simulink model "QuadcopterControl"  (R2026a)
settings: Solver=VariableStepAuto  StopTime=20
libraries: slpidlib x6, matrix_library x4
settings Model: SimulationMode=accelerator  Creator=nfrey  LastModifiedBy=nfrey
settings DataIOCC: InspectSignalLogs=on

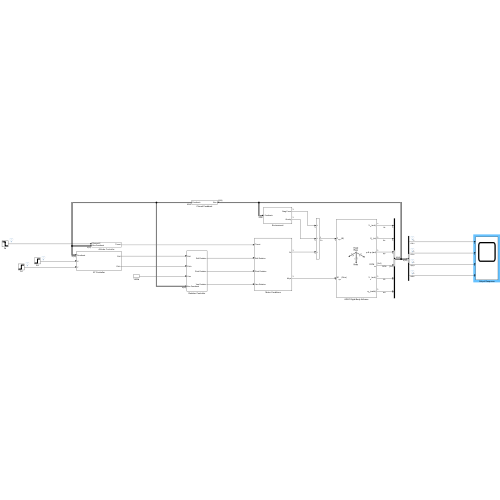
[thumbnail: Simulink's stored preview of the top-level diagram]
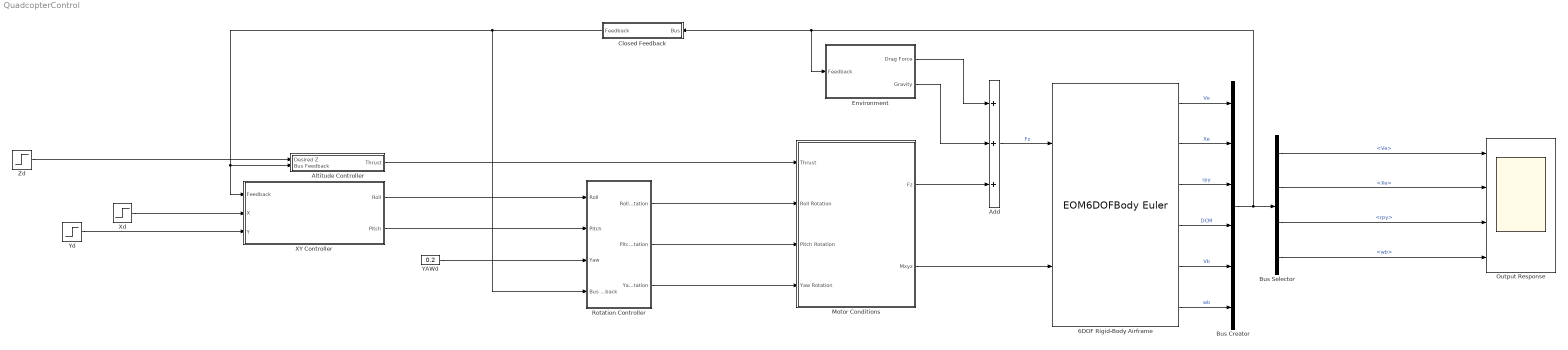
== system QuadcopterControl ==
  6DOF Rigid-Body Airframe : EOM6DOFBodyEuler
  Add : Sum  Inputs=+++
  Altitude Controller : Subsystem
  Bus Creator : BusCreator  Inputs=6
  Bus Selector : BusSelector  OutputSignals=Ve,Xe,rpy,wb
  Closed Feedback : Subsystem
  Environment : Subsystem
  Motor Conditions : Subsystem
  Output Response : Scope  NumInputPorts=4
      settings: ActiveDisplayYMinimum=-17.054653965110973  ActiveDisplayYMaximum=83.725752230949269
  Rotation Controller : Subsystem
  XY Controller : Subsystem
  Xd : Step  FinalValue=10  SampleTime=0
  YAWd : Constant  Value=0.2
  Yd : Step  FinalValue=5  SampleTime=0
  Zd : Step  FinalValue=-10  SampleTime=0
  wires:
  XY Controller/2(Pitch) -> Rotation Controller/2(Pitch)
  XY Controller/1(Roll) -> Rotation Controller/1(Roll)
  YAWd/1 -> Rotation Controller/3(Yaw)
  Bus Selector/3 -> Output Response/3  "<rpy>"
  Motor Conditions/1(Fz) -> Add/3
  Bus Selector/4 -> Output Response/4  "<wb>"
  Rotation Controller/2(Pitch Rotation) -> Motor Conditions/3(Pitch Rotation)
  Rotation Controller/3(Yaw Rotation) -> Motor Conditions/4(Yaw Rotation)
  Altitude Controller/1(Thrust) -> Motor Conditions/1(Thrust)
  Environment/1(Drag Force) -> Add/1
  Rotation Controller/1(Roll Rotation) -> Motor Conditions/2(Roll Rotation)
  Bus Selector/2 -> Output Response/2  "<Xe>"
  Bus Selector/1 -> Output Response/1  "<Ve>"
  6DOF Rigid-Body Airframe/2 -> Bus Creator/2  "Xe"
  6DOF Rigid-Body Airframe/4 -> Bus Creator/4  "DCM"
  6DOF Rigid-Body Airframe/1 -> Bus Creator/1  "Ve"
  6DOF Rigid-Body Airframe/3 -> Bus Creator/3  "rpy"
  6DOF Rigid-Body Airframe/6 -> Bus Creator/6  "wb"
  6DOF Rigid-Body Airframe/5 -> Bus Creator/5  "Vb"
  Bus Creator/1 -> Environment/1(" Feedback"), Closed Feedback/1(" Bus"), Bus Selector/1
  Environment/2(Gravity) -> Add/2
  Motor Conditions/2(Mxyz) -> 6DOF Rigid-Body Airframe/2
  Add/1 -> 6DOF Rigid-Body Airframe/1  "Fz"
  Closed Feedback/1(Feedback) -> Rotation Controller/4(Bus Feedback), XY Controller/1(Feedback), Altitude Controller/2(Bus Feedback)
  Xd/1 -> XY Controller/2(X)
  Yd/1 -> XY Controller/3(Y)
  Zd/1 -> Altitude Controller/1(Desired Z)

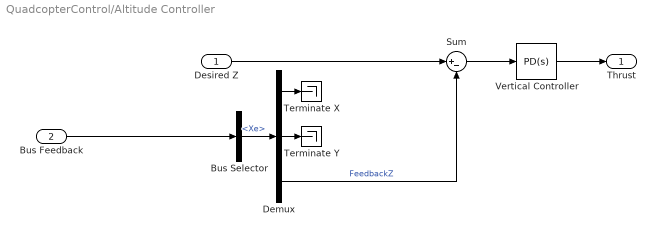
== system QuadcopterControl/Altitude Controller ==
  Desired Z : Inport
  Bus Feedback : Inport  Port=2
  Bus Selector : BusSelector  OutputSignals=Xe
  Demux : Demux  Outputs=3
  Sum : Sum  Inputs=|+-
  Terminate X : Terminator
  Terminate Y : Terminator
  Vertical Controller : slpidlib/PID Controller  Controller=PD  Form=Parallel  TimeDomain=Continuous-time  UseExternalTs=off  SampleTime=-1  IntegratorMethod=Forward Euler  FilterMethod=Forward Euler  ControllerParametersSource=internal  P=1.68756862780495  I=1  UseKiTs=off  D=2.04119632180359  UseExternalDerivativeSource=off  N=476.409993785113  UseFilter=on  TunerSelectOption=Transfer Function Based (PID Tuner App)  InitialConditionSource=internal  InitialConditionForIntegrator=0  InitialConditionForFilter=0  DifferentiatorICPrevScaledInput=0  ExternalReset=none  TrackingMode=off  Kt=1  LimitOutput=off  SatLimitsSource=internal  UpperSaturationLimit=inf  LowerSaturationLimit=-inf  LinearizeAsGain=on  AntiWindupMode=none  Kb=1  LimitIntegrator=off  UpperIntegratorSaturationLimit=inf  LowerIntegratorSaturationLimit=-inf  POutMin=[]  POutMax=[]  IOutMin=[]  IOutMax=[]  DOutMin=[]  DOutMax=[]  NOutMin=[]  NOutMax=[]  SumOutMin=[]  SumOutMax=[]  SaturationOutMin=[]  SaturationOutMax=[]  PParamMin=[]  PParamMax=[]  IParamMin=[]  IParamMax=[]  DParamMin=[]  DParamMax=[]  NParamMin=[]  NParamMax=[]  KbParamMin=[]  KbParamMax=[]  KtParamMin=[]  KtParamMax=[]  KbOutMin=[]  KbOutMax=[]  KtOutMin=[]  KtOutMax=[]  IntegratorOutMin=[]  IntegratorOutMax=[]  FilterOutMin=[]  FilterOutMax=[]  SumI1OutMin=[]  SumI1OutMax=[]  SumI2OutMin=[]  SumI2OutMax=[]  SumI3OutMin=[]  SumI3OutMax=[]  SumI4OutMin=[]  SumI4OutMax=[]  SumDOutMin=[]  SumDOutMax=[]  DifferentiatorOutMin=[]  DifferentiatorOutMax=[]  FilterDiffOutCoefMin=[]  FilterDiffOutCoefMax=[]  ReciprocalOutMin=[]  ReciprocalOutMax=[]  SumDenOutMin=[]  SumDenOutMax=[]  SumNumOutMin=[]  SumNumOutMax=[]  DivideOutMin=[]  DivideOutMax=[]  UdiffTsProdOutMin=[]  UdiffTsProdOutMax=[]  NTsProdOutMin=[]  NTsProdOutMax=[]  UintegralTsProdOutMin=[]  UintegralTsProdOutMax=[]  UngainTsProdOutMin=[]  UngainTsProdOutMax=[]  ClampingZeroOutDataTypeStr=Inherit: Inherit via back propagation  ClampingZeroOutMin=[]  ClampingZeroOutMax=[]  FilterDenConstantOutDataTypeStr=Inherit: Inherit via back propagation  FilterDenConstantOutMin=[]  FilterDenConstantOutMax=[]  PCopyOutDataTypeStr=Inherit: Inherit via back propagation  PCopyOutMin=[]  PCopyOutMax=[]  NCopyOutDataTypeStr=Inherit: Inherit via back propagation  NCopyOutMin=[]  NCopyOutMax=[]  IntegratorContinuousStateAttributes=''  IntegratorStateMustResolveToSignalObject=off  IntegratorRTWStateStorageClass=Auto  FilterContinuousStateAttributes=''  FilterStateMustResolveToSignalObject=off  FilterRTWStateStorageClass=Auto  ParallelPVariant=InternalParameters  IdealPVariant=Disabled  IVariant=Disabled  DVariant=InternalParameters  IntegratorVariant=Disabled  SatVariant=Disabled  AWVariant=Disabled  PCopyVariant=Disabled  TRVariant=Disabled  FdbkBlocksVariant=Forward  IdealPFdbkVariant=Disabled  SatFdbkVariant=Disabled  DerivativeFilterVariant=ContFilter  NVariant=InternalParameters  NCopyVariant=Disabled  FilterICVariant=InternalICsFilter  IntegratorICVariant=Disabled  ExternalResetVariant=Disabled  TRSumVariant=Passthrough  SumFdbkVariant=Disabled  SumVariant=Sum_PD  TsampFilterVariant=InternalTs  TsampNgainVariant=Passthrough  TsampIntegralVariant=Disabled_SignalSpec  ExternalSaturationOutDataTypeStr=Inherit: Same as second input  DerivativeSourceVariant=ErrorSignal  PreIntVariant=InternalPreInt
  Thrust : Outport
  wires:
  Bus Feedback/1 -> Bus Selector/1
  Bus Selector/1 -> Demux/1  "<Xe>"
  Demux/1 -> Terminate X/1
  Demux/2 -> Terminate Y/1
  Desired Z/1 -> Sum/1
  Demux/3 -> Sum/2  "FeedbackZ"
  Sum/1 -> Vertical Controller/1
  Vertical Controller/1 -> Thrust/1

== system QuadcopterControl/Closed Feedback ==
  " Bus" : Inport
  Feedback : Outport
  wires:
  " Bus"/1 -> Feedback/1

== system QuadcopterControl/Environment ==
  " Feedback" : Inport
  Drag : Subsystem
  Gravity Variable : Subsystem
  Drag Force : Outport
  Gravity : Outport  Port=2
  wires:
  " Feedback"/1 -> Gravity Variable/1(In1), Drag/1(In1)
  Drag/1(Drag Force) -> Drag Force/1
  Gravity Variable/1(Gravity) -> Gravity/1

== system QuadcopterControl/Motor Conditions ==
  Thrust : Inport
  Roll Rotation : Inport  Port=2
  Pitch Rotation : Inport  Port=3
  Yaw Rotation : Inport  Port=4
  Moment & Net Force : Subsystem
  Rotor Correction : Subsystem
  Fz : Outport
  Mxyz : Outport  Port=2
  wires:
  Roll Rotation/1 -> Rotor Correction/2(Roll)
  Rotor Correction/1(Propeller Velocity) -> Moment & Net Force/1(Propeller Velocity)
  Moment & Net Force/1(OutputFz) -> Fz/1
  Pitch Rotation/1 -> Rotor Correction/3(Pitch)
  Thrust/1 -> Rotor Correction/1(Thrust)
  Moment & Net Force/2(Moment) -> Mxyz/1
  Yaw Rotation/1 -> Rotor Correction/4(Yaw)

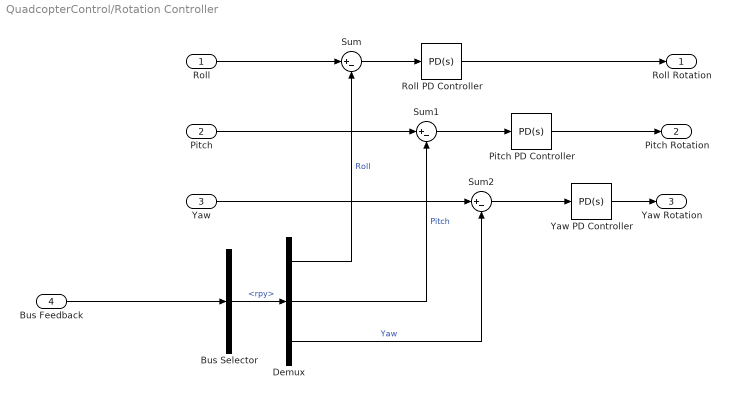
== system QuadcopterControl/Rotation Controller ==
  Roll : Inport
  Pitch : Inport  Port=2
  Yaw : Inport  Port=3
  Bus Feedback : Inport  Port=4
  Bus Selector : BusSelector  OutputSignals=rpy
  Demux : Demux  Outputs=3
  Pitch PD Controller : slpidlib/PID Controller  Controller=PD  Form=Parallel  TimeDomain=Continuous-time  UseExternalTs=off  SampleTime=-1  IntegratorMethod=Forward Euler  FilterMethod=Forward Euler  ControllerParametersSource=internal  P=.684  I=1  UseKiTs=off  D=1.41  UseExternalDerivativeSource=off  N=100  UseFilter=on  TunerSelectOption=Transfer Function Based (PID Tuner App)  InitialConditionSource=internal  InitialConditionForIntegrator=0  InitialConditionForFilter=0  DifferentiatorICPrevScaledInput=0  ExternalReset=none  TrackingMode=off  Kt=1  LimitOutput=off  SatLimitsSource=internal  UpperSaturationLimit=inf  LowerSaturationLimit=-inf  LinearizeAsGain=on  AntiWindupMode=none  Kb=1  LimitIntegrator=off  UpperIntegratorSaturationLimit=inf  LowerIntegratorSaturationLimit=-inf  POutMin=[]  POutMax=[]  IOutMin=[]  IOutMax=[]  DOutMin=[]  DOutMax=[]  NOutMin=[]  NOutMax=[]  SumOutMin=[]  SumOutMax=[]  SaturationOutMin=[]  SaturationOutMax=[]  PParamMin=[]  PParamMax=[]  IParamMin=[]  IParamMax=[]  DParamMin=[]  DParamMax=[]  NParamMin=[]  NParamMax=[]  KbParamMin=[]  KbParamMax=[]  KtParamMin=[]  KtParamMax=[]  KbOutMin=[]  KbOutMax=[]  KtOutMin=[]  KtOutMax=[]  IntegratorOutMin=[]  IntegratorOutMax=[]  FilterOutMin=[]  FilterOutMax=[]  SumI1OutMin=[]  SumI1OutMax=[]  SumI2OutMin=[]  SumI2OutMax=[]  SumI3OutMin=[]  SumI3OutMax=[]  SumI4OutMin=[]  SumI4OutMax=[]  SumDOutMin=[]  SumDOutMax=[]  DifferentiatorOutMin=[]  DifferentiatorOutMax=[]  FilterDiffOutCoefMin=[]  FilterDiffOutCoefMax=[]  ReciprocalOutMin=[]  ReciprocalOutMax=[]  SumDenOutMin=[]  SumDenOutMax=[]  SumNumOutMin=[]  SumNumOutMax=[]  DivideOutMin=[]  DivideOutMax=[]  UdiffTsProdOutMin=[]  UdiffTsProdOutMax=[]  NTsProdOutMin=[]  NTsProdOutMax=[]  UintegralTsProdOutMin=[]  UintegralTsProdOutMax=[]  UngainTsProdOutMin=[]  UngainTsProdOutMax=[]  ClampingZeroOutDataTypeStr=Inherit: Inherit via back propagation  ClampingZeroOutMin=[]  ClampingZeroOutMax=[]  FilterDenConstantOutDataTypeStr=Inherit: Inherit via back propagation  FilterDenConstantOutMin=[]  FilterDenConstantOutMax=[]  PCopyOutDataTypeStr=Inherit: Inherit via back propagation  PCopyOutMin=[]  PCopyOutMax=[]  NCopyOutDataTypeStr=Inherit: Inherit via back propagation  NCopyOutMin=[]  NCopyOutMax=[]  IntegratorContinuousStateAttributes=''  IntegratorStateMustResolveToSignalObject=off  IntegratorRTWStateStorageClass=Auto  FilterContinuousStateAttributes=''  FilterStateMustResolveToSignalObject=off  FilterRTWStateStorageClass=Auto  ParallelPVariant=InternalParameters  IdealPVariant=Disabled  IVariant=Disabled  DVariant=InternalParameters  IntegratorVariant=Disabled  SatVariant=Disabled  AWVariant=Disabled  PCopyVariant=Disabled  TRVariant=Disabled  FdbkBlocksVariant=Forward  IdealPFdbkVariant=Disabled  SatFdbkVariant=Disabled  DerivativeFilterVariant=ContFilter  NVariant=InternalParameters  NCopyVariant=Disabled  FilterICVariant=InternalICsFilter  IntegratorICVariant=Disabled  ExternalResetVariant=Disabled  TRSumVariant=Passthrough  SumFdbkVariant=Disabled  SumVariant=Sum_PD  TsampFilterVariant=InternalTs  TsampNgainVariant=Passthrough  TsampIntegralVariant=Disabled_SignalSpec  ExternalSaturationOutDataTypeStr=Inherit: Same as second input  DerivativeSourceVariant=ErrorSignal  PreIntVariant=InternalPreInt
  Roll PD Controller : slpidlib/PID Controller  Controller=PD  Form=Parallel  TimeDomain=Continuous-time  UseExternalTs=off  SampleTime=-1  IntegratorMethod=Forward Euler  FilterMethod=Forward Euler  ControllerParametersSource=internal  P=.684  I=1  UseKiTs=off  D=1.41  UseExternalDerivativeSource=off  N=100  UseFilter=on  TunerSelectOption=Transfer Function Based (PID Tuner App)  InitialConditionSource=internal  InitialConditionForIntegrator=0  InitialConditionForFilter=0  DifferentiatorICPrevScaledInput=0  ExternalReset=none  TrackingMode=off  Kt=1  LimitOutput=off  SatLimitsSource=internal  UpperSaturationLimit=inf  LowerSaturationLimit=-inf  LinearizeAsGain=on  AntiWindupMode=none  Kb=1  LimitIntegrator=off  UpperIntegratorSaturationLimit=inf  LowerIntegratorSaturationLimit=-inf  POutMin=[]  POutMax=[]  IOutMin=[]  IOutMax=[]  DOutMin=[]  DOutMax=[]  NOutMin=[]  NOutMax=[]  SumOutMin=[]  SumOutMax=[]  SaturationOutMin=[]  SaturationOutMax=[]  PParamMin=[]  PParamMax=[]  IParamMin=[]  IParamMax=[]  DParamMin=[]  DParamMax=[]  NParamMin=[]  NParamMax=[]  KbParamMin=[]  KbParamMax=[]  KtParamMin=[]  KtParamMax=[]  KbOutMin=[]  KbOutMax=[]  KtOutMin=[]  KtOutMax=[]  IntegratorOutMin=[]  IntegratorOutMax=[]  FilterOutMin=[]  FilterOutMax=[]  SumI1OutMin=[]  SumI1OutMax=[]  SumI2OutMin=[]  SumI2OutMax=[]  SumI3OutMin=[]  SumI3OutMax=[]  SumI4OutMin=[]  SumI4OutMax=[]  SumDOutMin=[]  SumDOutMax=[]  DifferentiatorOutMin=[]  DifferentiatorOutMax=[]  FilterDiffOutCoefMin=[]  FilterDiffOutCoefMax=[]  ReciprocalOutMin=[]  ReciprocalOutMax=[]  SumDenOutMin=[]  SumDenOutMax=[]  SumNumOutMin=[]  SumNumOutMax=[]  DivideOutMin=[]  DivideOutMax=[]  UdiffTsProdOutMin=[]  UdiffTsProdOutMax=[]  NTsProdOutMin=[]  NTsProdOutMax=[]  UintegralTsProdOutMin=[]  UintegralTsProdOutMax=[]  UngainTsProdOutMin=[]  UngainTsProdOutMax=[]  ClampingZeroOutDataTypeStr=Inherit: Inherit via back propagation  ClampingZeroOutMin=[]  ClampingZeroOutMax=[]  FilterDenConstantOutDataTypeStr=Inherit: Inherit via back propagation  FilterDenConstantOutMin=[]  FilterDenConstantOutMax=[]  PCopyOutDataTypeStr=Inherit: Inherit via back propagation  PCopyOutMin=[]  PCopyOutMax=[]  NCopyOutDataTypeStr=Inherit: Inherit via back propagation  NCopyOutMin=[]  NCopyOutMax=[]  IntegratorContinuousStateAttributes=''  IntegratorStateMustResolveToSignalObject=off  IntegratorRTWStateStorageClass=Auto  FilterContinuousStateAttributes=''  FilterStateMustResolveToSignalObject=off  FilterRTWStateStorageClass=Auto  ParallelPVariant=InternalParameters  IdealPVariant=Disabled  IVariant=Disabled  DVariant=InternalParameters  IntegratorVariant=Disabled  SatVariant=Disabled  AWVariant=Disabled  PCopyVariant=Disabled  TRVariant=Disabled  FdbkBlocksVariant=Forward  IdealPFdbkVariant=Disabled  SatFdbkVariant=Disabled  DerivativeFilterVariant=ContFilter  NVariant=InternalParameters  NCopyVariant=Disabled  FilterICVariant=InternalICsFilter  IntegratorICVariant=Disabled  ExternalResetVariant=Disabled  TRSumVariant=Passthrough  SumFdbkVariant=Disabled  SumVariant=Sum_PD  TsampFilterVariant=InternalTs  TsampNgainVariant=Passthrough  TsampIntegralVariant=Disabled_SignalSpec  ExternalSaturationOutDataTypeStr=Inherit: Same as second input  DerivativeSourceVariant=ErrorSignal  PreIntVariant=InternalPreInt
  Sum : Sum  Inputs=|+-
  Sum1 : Sum  Inputs=|+-
  Sum2 : Sum  Inputs=|+-
  Yaw PD Controller : slpidlib/PID Controller  Controller=PD  Form=Parallel  TimeDomain=Continuous-time  UseExternalTs=off  SampleTime=-1  IntegratorMethod=Forward Euler  FilterMethod=Forward Euler  ControllerParametersSource=internal  P=0.684167402629352  I=1  UseKiTs=off  D=1.4072621028923  UseExternalDerivativeSource=off  N=100  UseFilter=on  TunerSelectOption=Transfer Function Based (PID Tuner App)  InitialConditionSource=internal  InitialConditionForIntegrator=0  InitialConditionForFilter=0  DifferentiatorICPrevScaledInput=0  ExternalReset=none  TrackingMode=off  Kt=1  LimitOutput=off  SatLimitsSource=internal  UpperSaturationLimit=inf  LowerSaturationLimit=-inf  LinearizeAsGain=on  AntiWindupMode=none  Kb=1  LimitIntegrator=off  UpperIntegratorSaturationLimit=inf  LowerIntegratorSaturationLimit=-inf  POutMin=[]  POutMax=[]  IOutMin=[]  IOutMax=[]  DOutMin=[]  DOutMax=[]  NOutMin=[]  NOutMax=[]  SumOutMin=[]  SumOutMax=[]  SaturationOutMin=[]  SaturationOutMax=[]  PParamMin=[]  PParamMax=[]  IParamMin=[]  IParamMax=[]  DParamMin=[]  DParamMax=[]  NParamMin=[]  NParamMax=[]  KbParamMin=[]  KbParamMax=[]  KtParamMin=[]  KtParamMax=[]  KbOutMin=[]  KbOutMax=[]  KtOutMin=[]  KtOutMax=[]  IntegratorOutMin=[]  IntegratorOutMax=[]  FilterOutMin=[]  FilterOutMax=[]  SumI1OutMin=[]  SumI1OutMax=[]  SumI2OutMin=[]  SumI2OutMax=[]  SumI3OutMin=[]  SumI3OutMax=[]  SumI4OutMin=[]  SumI4OutMax=[]  SumDOutMin=[]  SumDOutMax=[]  DifferentiatorOutMin=[]  DifferentiatorOutMax=[]  FilterDiffOutCoefMin=[]  FilterDiffOutCoefMax=[]  ReciprocalOutMin=[]  ReciprocalOutMax=[]  SumDenOutMin=[]  SumDenOutMax=[]  SumNumOutMin=[]  SumNumOutMax=[]  DivideOutMin=[]  DivideOutMax=[]  UdiffTsProdOutMin=[]  UdiffTsProdOutMax=[]  NTsProdOutMin=[]  NTsProdOutMax=[]  UintegralTsProdOutMin=[]  UintegralTsProdOutMax=[]  UngainTsProdOutMin=[]  UngainTsProdOutMax=[]  ClampingZeroOutDataTypeStr=Inherit: Inherit via back propagation  ClampingZeroOutMin=[]  ClampingZeroOutMax=[]  FilterDenConstantOutDataTypeStr=Inherit: Inherit via back propagation  FilterDenConstantOutMin=[]  FilterDenConstantOutMax=[]  PCopyOutDataTypeStr=Inherit: Inherit via back propagation  PCopyOutMin=[]  PCopyOutMax=[]  NCopyOutDataTypeStr=Inherit: Inherit via back propagation  NCopyOutMin=[]  NCopyOutMax=[]  IntegratorContinuousStateAttributes=''  IntegratorStateMustResolveToSignalObject=off  IntegratorRTWStateStorageClass=Auto  FilterContinuousStateAttributes=''  FilterStateMustResolveToSignalObject=off  FilterRTWStateStorageClass=Auto  ParallelPVariant=InternalParameters  IdealPVariant=Disabled  IVariant=Disabled  DVariant=InternalParameters  IntegratorVariant=Disabled  SatVariant=Disabled  AWVariant=Disabled  PCopyVariant=Disabled  TRVariant=Disabled  FdbkBlocksVariant=Forward  IdealPFdbkVariant=Disabled  SatFdbkVariant=Disabled  DerivativeFilterVariant=ContFilter  NVariant=InternalParameters  NCopyVariant=Disabled  FilterICVariant=InternalICsFilter  IntegratorICVariant=Disabled  ExternalResetVariant=Disabled  TRSumVariant=Passthrough  SumFdbkVariant=Disabled  SumVariant=Sum_PD  TsampFilterVariant=InternalTs  TsampNgainVariant=Passthrough  TsampIntegralVariant=Disabled_SignalSpec  ExternalSaturationOutDataTypeStr=Inherit: Same as second input  DerivativeSourceVariant=ErrorSignal  PreIntVariant=InternalPreInt
  Roll Rotation : Outport
  Pitch Rotation : Outport  Port=2
  Yaw Rotation : Outport  Port=3
  wires:
  Bus Feedback/1 -> Bus Selector/1
  Bus Selector/1 -> Demux/1  "<rpy>"
  Roll/1 -> Sum/1
  Sum/1 -> Roll PD Controller/1
  Sum1/1 -> Pitch PD Controller/1
  Pitch/1 -> Sum1/1
  Yaw/1 -> Sum2/1
  Sum2/1 -> Yaw PD Controller/1
  Roll PD Controller/1 -> Roll Rotation/1
  Pitch PD Controller/1 -> Pitch Rotation/1
  Yaw PD Controller/1 -> Yaw Rotation/1
  Demux/1 -> Sum/2  "Roll"
  Demux/2 -> Sum1/2  "Pitch"
  Demux/3 -> Sum2/2  "Yaw"

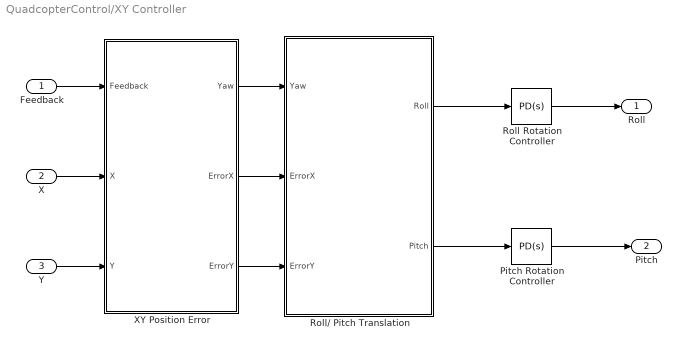
== system QuadcopterControl/XY Controller ==
  Feedback : Inport
  X : Inport  Port=2
  Y : Inport  Port=3
  Pitch Rotation Controller : slpidlib/PID Controller  Controller=PD  Form=Parallel  TimeDomain=Continuous-time  UseExternalTs=off  SampleTime=-1  IntegratorMethod=Forward Euler  FilterMethod=Forward Euler  ControllerParametersSource=internal  P=0.02  I=1  UseKiTs=off  D=0.15  UseExternalDerivativeSource=off  N=170  UseFilter=on  TunerSelectOption=Transfer Function Based (PID Tuner App)  InitialConditionSource=internal  InitialConditionForIntegrator=0  InitialConditionForFilter=0  DifferentiatorICPrevScaledInput=0  ExternalReset=none  TrackingMode=off  Kt=1  LimitOutput=on  SatLimitsSource=internal  UpperSaturationLimit=0.25  LowerSaturationLimit=-0.25  LinearizeAsGain=on  AntiWindupMode=none  Kb=1  LimitIntegrator=off  UpperIntegratorSaturationLimit=inf  LowerIntegratorSaturationLimit=-inf  POutMin=[]  POutMax=[]  IOutMin=[]  IOutMax=[]  DOutMin=[]  DOutMax=[]  NOutMin=[]  NOutMax=[]  SumOutMin=[]  SumOutMax=[]  SaturationOutMin=[]  SaturationOutMax=[]  PParamMin=[]  PParamMax=[]  IParamMin=[]  IParamMax=[]  DParamMin=[]  DParamMax=[]  NParamMin=[]  NParamMax=[]  KbParamMin=[]  KbParamMax=[]  KtParamMin=[]  KtParamMax=[]  KbOutMin=[]  KbOutMax=[]  KtOutMin=[]  KtOutMax=[]  IntegratorOutMin=[]  IntegratorOutMax=[]  FilterOutMin=[]  FilterOutMax=[]  SumI1OutMin=[]  SumI1OutMax=[]  SumI2OutMin=[]  SumI2OutMax=[]  SumI3OutMin=[]  SumI3OutMax=[]  SumI4OutMin=[]  SumI4OutMax=[]  SumDOutMin=[]  SumDOutMax=[]  DifferentiatorOutMin=[]  DifferentiatorOutMax=[]  FilterDiffOutCoefMin=[]  FilterDiffOutCoefMax=[]  ReciprocalOutMin=[]  ReciprocalOutMax=[]  SumDenOutMin=[]  SumDenOutMax=[]  SumNumOutMin=[]  SumNumOutMax=[]  DivideOutMin=[]  DivideOutMax=[]  UdiffTsProdOutMin=[]  UdiffTsProdOutMax=[]  NTsProdOutMin=[]  NTsProdOutMax=[]  UintegralTsProdOutMin=[]  UintegralTsProdOutMax=[]  UngainTsProdOutMin=[]  UngainTsProdOutMax=[]  ClampingZeroOutDataTypeStr=Inherit: Inherit via back propagation  ClampingZeroOutMin=[]  ClampingZeroOutMax=[]  FilterDenConstantOutDataTypeStr=Inherit: Inherit via back propagation  FilterDenConstantOutMin=[]  FilterDenConstantOutMax=[]  PCopyOutDataTypeStr=Inherit: Inherit via back propagation  PCopyOutMin=[]  PCopyOutMax=[]  NCopyOutDataTypeStr=Inherit: Inherit via back propagation  NCopyOutMin=[]  NCopyOutMax=[]  IntegratorContinuousStateAttributes=''  IntegratorStateMustResolveToSignalObject=off  IntegratorRTWStateStorageClass=Auto  FilterContinuousStateAttributes=''  FilterStateMustResolveToSignalObject=off  FilterRTWStateStorageClass=Auto  ParallelPVariant=InternalParameters  IdealPVariant=Disabled  IVariant=Disabled  DVariant=InternalParameters  IntegratorVariant=Disabled  SatVariant=Enabled  AWVariant=Disabled  PCopyVariant=Disabled  TRVariant=Disabled  FdbkBlocksVariant=Forward  IdealPFdbkVariant=Disabled  SatFdbkVariant=Disabled  DerivativeFilterVariant=ContFilter  NVariant=InternalParameters  NCopyVariant=Disabled  FilterICVariant=InternalICsFilter  IntegratorICVariant=Disabled  ExternalResetVariant=Disabled  TRSumVariant=Passthrough  SumFdbkVariant=Disabled  SumVariant=Sum_PD  TsampFilterVariant=InternalTs  TsampNgainVariant=Passthrough  TsampIntegralVariant=Disabled_SignalSpec  ExternalSaturationOutDataTypeStr=Inherit: Same as second input  DerivativeSourceVariant=ErrorSignal  PreIntVariant=InternalPreInt
  Roll Rotation Controller : slpidlib/PID Controller  Controller=PD  Form=Parallel  TimeDomain=Continuous-time  UseExternalTs=off  SampleTime=-1  IntegratorMethod=Forward Euler  FilterMethod=Forward Euler  ControllerParametersSource=internal  P=0.02  I=1  UseKiTs=off  D=0.15  UseExternalDerivativeSource=off  N=170  UseFilter=on  TunerSelectOption=Transfer Function Based (PID Tuner App)  InitialConditionSource=internal  InitialConditionForIntegrator=0  InitialConditionForFilter=0  DifferentiatorICPrevScaledInput=0  ExternalReset=none  TrackingMode=off  Kt=1  LimitOutput=on  SatLimitsSource=internal  UpperSaturationLimit=.25  LowerSaturationLimit=-.25  LinearizeAsGain=on  AntiWindupMode=none  Kb=1  LimitIntegrator=off  UpperIntegratorSaturationLimit=inf  LowerIntegratorSaturationLimit=-inf  POutMin=[]  POutMax=[]  IOutMin=[]  IOutMax=[]  DOutMin=[]  DOutMax=[]  NOutMin=[]  NOutMax=[]  SumOutMin=[]  SumOutMax=[]  SaturationOutMin=[]  SaturationOutMax=[]  PParamMin=[]  PParamMax=[]  IParamMin=[]  IParamMax=[]  DParamMin=[]  DParamMax=[]  NParamMin=[]  NParamMax=[]  KbParamMin=[]  KbParamMax=[]  KtParamMin=[]  KtParamMax=[]  KbOutMin=[]  KbOutMax=[]  KtOutMin=[]  KtOutMax=[]  IntegratorOutMin=[]  IntegratorOutMax=[]  FilterOutMin=[]  FilterOutMax=[]  SumI1OutMin=[]  SumI1OutMax=[]  SumI2OutMin=[]  SumI2OutMax=[]  SumI3OutMin=[]  SumI3OutMax=[]  SumI4OutMin=[]  SumI4OutMax=[]  SumDOutMin=[]  SumDOutMax=[]  DifferentiatorOutMin=[]  DifferentiatorOutMax=[]  FilterDiffOutCoefMin=[]  FilterDiffOutCoefMax=[]  ReciprocalOutMin=[]  ReciprocalOutMax=[]  SumDenOutMin=[]  SumDenOutMax=[]  SumNumOutMin=[]  SumNumOutMax=[]  DivideOutMin=[]  DivideOutMax=[]  UdiffTsProdOutMin=[]  UdiffTsProdOutMax=[]  NTsProdOutMin=[]  NTsProdOutMax=[]  UintegralTsProdOutMin=[]  UintegralTsProdOutMax=[]  UngainTsProdOutMin=[]  UngainTsProdOutMax=[]  ClampingZeroOutDataTypeStr=Inherit: Inherit via back propagation  ClampingZeroOutMin=[]  ClampingZeroOutMax=[]  FilterDenConstantOutDataTypeStr=Inherit: Inherit via back propagation  FilterDenConstantOutMin=[]  FilterDenConstantOutMax=[]  PCopyOutDataTypeStr=Inherit: Inherit via back propagation  PCopyOutMin=[]  PCopyOutMax=[]  NCopyOutDataTypeStr=Inherit: Inherit via back propagation  NCopyOutMin=[]  NCopyOutMax=[]  IntegratorContinuousStateAttributes=''  IntegratorStateMustResolveToSignalObject=off  IntegratorRTWStateStorageClass=Auto  FilterContinuousStateAttributes=''  FilterStateMustResolveToSignalObject=off  FilterRTWStateStorageClass=Auto  ParallelPVariant=InternalParameters  IdealPVariant=Disabled  IVariant=Disabled  DVariant=InternalParameters  IntegratorVariant=Disabled  SatVariant=Enabled  AWVariant=Disabled  PCopyVariant=Disabled  TRVariant=Disabled  FdbkBlocksVariant=Forward  IdealPFdbkVariant=Disabled  SatFdbkVariant=Disabled  DerivativeFilterVariant=ContFilter  NVariant=InternalParameters  NCopyVariant=Disabled  FilterICVariant=InternalICsFilter  IntegratorICVariant=Disabled  ExternalResetVariant=Disabled  TRSumVariant=Passthrough  SumFdbkVariant=Disabled  SumVariant=Sum_PD  TsampFilterVariant=InternalTs  TsampNgainVariant=Passthrough  TsampIntegralVariant=Disabled_SignalSpec  ExternalSaturationOutDataTypeStr=Inherit: Same as second input  DerivativeSourceVariant=ErrorSignal  PreIntVariant=InternalPreInt
  Roll/ Pitch Translation : Subsystem
  XY Position Error : Subsystem
  Roll : Outport
  Pitch : Outport  Port=2
  wires:
  Feedback/1 -> XY Position Error/1(Feedback)
  X/1 -> XY Position Error/2(X)
  Y/1 -> XY Position Error/3(Y)
  XY Position Error/1(Yaw) -> Roll/ Pitch Translation/1(Yaw)
  XY Position Error/2(ErrorX) -> Roll/ Pitch Translation/2(ErrorX)
  XY Position Error/3(ErrorY) -> Roll/ Pitch Translation/3(ErrorY)
  Pitch Rotation Controller/1 -> Pitch/1
  Roll/ Pitch Translation/2(Pitch) -> Pitch Rotation Controller/1
  Roll/ Pitch Translation/1(Roll) -> Roll Rotation Controller/1
  Roll Rotation Controller/1 -> Roll/1

== system QuadcopterControl/Environment/Drag ==
  In1 : Inport
  Bus Selector : BusSelector  OutputSignals=Vb
  Dot Product : DotProduct  OutDataTypeStr=Inherit: Inherit via internal rule
  Drag Gain : Gain  Gain=-0.005
  Product : Product
  Sqrt : Sqrt
  Drag Force : Outport
  wires:
  In1/1 -> Bus Selector/1
  Bus Selector/1 -> Dot Product/1, Product/2, Dot Product/2  "<Vb>"
  Dot Product/1 -> Sqrt/1
  Sqrt/1 -> Product/1
  Product/1 -> Drag Gain/1
  Drag Gain/1 -> Drag Force/1

== system QuadcopterControl/Environment/Gravity Variable ==
  In1 : Inport
  Gravity Acceleration : Subsystem
  Mass : Gain
  Gravity : Outport
  wires:
  Gravity Acceleration/1(Out1) -> Mass/1
  Mass/1 -> Gravity/1
  In1/1 -> Gravity Acceleration/1(In1)

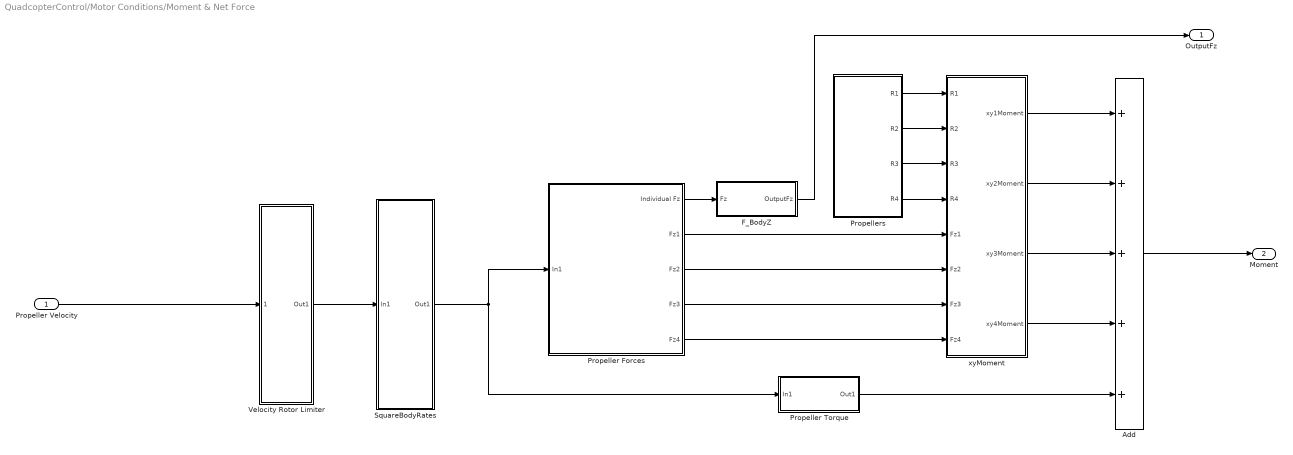
== system QuadcopterControl/Motor Conditions/Moment & Net Force ==
  Propeller Velocity : Inport
  Add : Sum  Inputs=+++++
  F_BodyZ : Subsystem
  Propeller Forces : Subsystem
  "Propeller Torque " : Subsystem
  Propellers : Subsystem
  SquareBodyRates : Subsystem
  Velocity Rotor Limiter : Subsystem
  xyMoment : Subsystem
  OutputFz : Outport
  Moment : Outport  Port=2
  wires:
  Add/1 -> Moment/1
  F_BodyZ/1(OutputFz) -> OutputFz/1
  Propeller Velocity/1 -> Velocity Rotor Limiter/1(Propeller Velocity)
  Propeller Forces/5(Fz4) -> xyMoment/8(Fz4)
  Propeller Forces/4(Fz3) -> xyMoment/7(Fz3)
  Propeller Forces/3(Fz2) -> xyMoment/6(Fz2)
  Propeller Forces/2(Fz1) -> xyMoment/5(Fz1)
  Propellers/4(R4) -> xyMoment/4(R4)
  Propellers/3(R3) -> xyMoment/3(R3)
  Propellers/2(R2) -> xyMoment/2(R2)
  Propellers/1(R1) -> xyMoment/1(R1)
  Propeller Forces/1(Individual Fz) -> F_BodyZ/1(Fz)
  xyMoment/1(xy1Moment) -> Add/1
  xyMoment/2(xy2Moment) -> Add/2
  xyMoment/3(xy3Moment) -> Add/3
  xyMoment/4(xy4Moment) -> Add/4
  "Propeller Torque "/1(Out1) -> Add/5
  SquareBodyRates/1(Out1) -> "Propeller Torque "/1(In1), Propeller Forces/1(In1)
  Velocity Rotor Limiter/1(Out1) -> SquareBodyRates/1(In1)

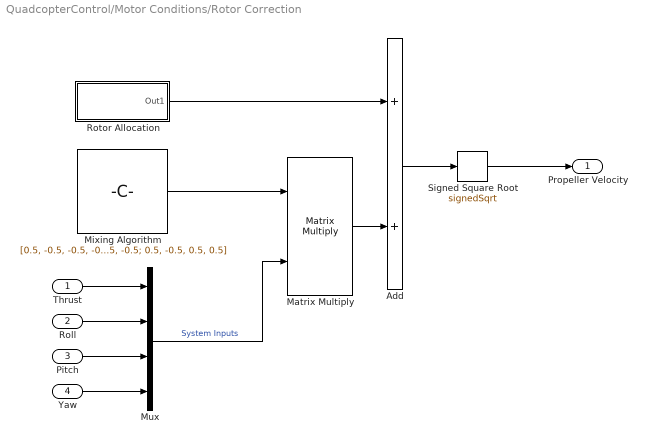
== system QuadcopterControl/Motor Conditions/Rotor Correction ==
  Thrust : Inport
  Roll : Inport  Port=2
  Pitch : Inport  Port=3
  Yaw : Inport  Port=4
  Add : Sum
  Matrix Multiply : Product  Multiplication=Matrix(*)
  Mixing Algorithm : Constant  Value="[0.5, -0.5, -0.5, -0.5 ; 0.5, 0.5, -0.5, 0.5 ;  0.5, 0.5, 0.5, -0.5; 0.5, -0.5, 0.5, 0.5]"  VectorParams1D=off
  Mux : Mux
  Rotor Allocation : Subsystem
  Signed Square Root : Sqrt  Operator=signedSqrt
  Propeller Velocity : Outport
  wires:
  Yaw/1 -> Mux/4
  Pitch/1 -> Mux/3
  Roll/1 -> Mux/2
  Thrust/1 -> Mux/1
  Mux/1 -> Matrix Multiply/2  "System Inputs"
  Mixing Algorithm/1 -> Matrix Multiply/1
  Matrix Multiply/1 -> Add/2
  Rotor Allocation/1(Out1) -> Add/1
  Add/1 -> Signed Square Root/1
  Signed Square Root/1 -> Propeller Velocity/1

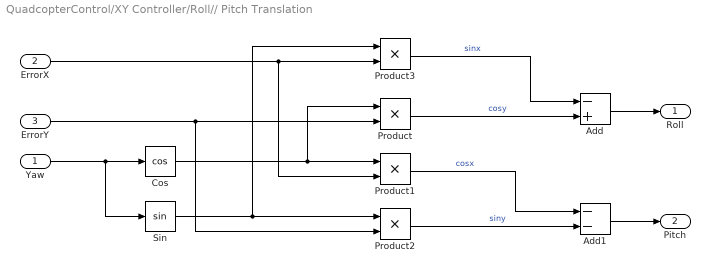
== system QuadcopterControl/XY Controller/Roll// Pitch Translation ==
  Yaw : Inport
  ErrorX : Inport  Port=2
  ErrorY : Inport  Port=3
  Add : Sum  Inputs=-+
  Add1 : Sum  Inputs=--
  Cos : Trigonometry  Operator=cos
  Product{,1..3} (4 alike) : Product
  Sin : Trigonometry
  Roll : Outport
  Pitch : Outport  Port=2
  wires:
  Add/1 -> Roll/1
  Add1/1 -> Pitch/1
  Yaw/1 -> Cos/1, Sin/1
  Cos/1 -> Product1/1, Product/1
  Sin/1 -> Product3/1, Product2/1
  ErrorX/1 -> Product1/2, Product3/2
  ErrorY/1 -> Product2/2, Product/2
  Product3/1 -> Add/1  "sinx"
  Product/1 -> Add/2  "cosy"
  Product2/1 -> Add1/2  "siny"
  Product1/1 -> Add1/1  "cosx"

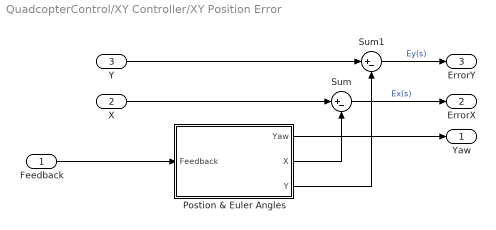
== system QuadcopterControl/XY Controller/XY Position Error ==
  Feedback : Inport
  X : Inport  Port=2
  Y : Inport  Port=3
  "Postion & Euler Angles " : Subsystem
  Sum : Sum  Inputs=|+-
  Sum1 : Sum  Inputs=|+-
  Yaw : Outport
  ErrorX : Outport  Port=2
  ErrorY : Outport  Port=3
  wires:
  Feedback/1 -> "Postion & Euler Angles "/1(Feedback)
  "Postion & Euler Angles "/1(Yaw) -> Yaw/1
  "Postion & Euler Angles "/2(X) -> Sum/2
  "Postion & Euler Angles "/3(Y) -> Sum1/2
  Sum1/1 -> ErrorY/1  "Ey(s)"
  Sum/1 -> ErrorX/1  "Ex(s)"
  X/1 -> Sum/1
  Y/1 -> Sum1/1

== system QuadcopterControl/Environment/Gravity Variable/Gravity Acceleration ==
  In1 : Inport
  Bus Selector : BusSelector  OutputSignals=DCM
  Gravity Z : Constant  Value=[0; 0; 9.81]
  Matrix Multiply : Product  Multiplication=Matrix(*)
  Out1 : Outport
  wires:
  In1/1 -> Bus Selector/1
  Gravity Z/1 -> Matrix Multiply/2
  Bus Selector/1 -> Matrix Multiply/1  "<DCM>"
  Matrix Multiply/1 -> Out1/1

== system QuadcopterControl/Motor Conditions/Moment & Net Force/F_BodyZ ==
  Fz : Inport
  Sum of Elements : Sum  Inputs=+
  vecZ : Subsystem
  OutputFz : Outport
  wires:
  Fz/1 -> Sum of Elements/1
  Sum of Elements/1 -> vecZ/1(InputFz)
  vecZ/1(OutputFz) -> OutputFz/1

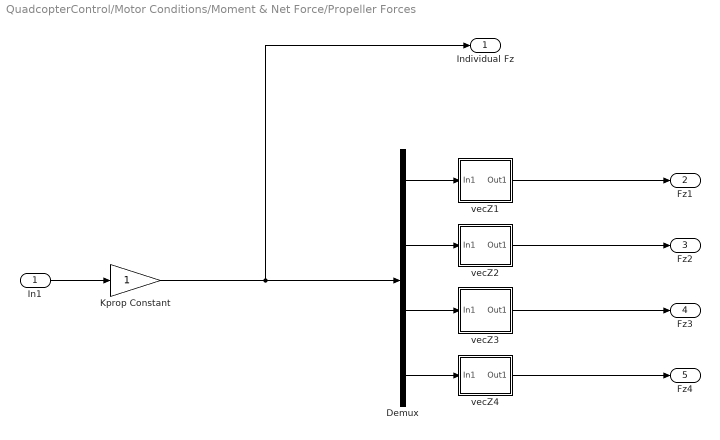
== system QuadcopterControl/Motor Conditions/Moment & Net Force/Propeller Forces ==
  In1 : Inport
  Demux : Demux
  Kprop Constant : Gain
  vecZ1 : Subsystem
  vecZ2 : Subsystem
  vecZ3 : Subsystem
  vecZ4 : Subsystem
  Individual Fz : Outport
  Fz1 : Outport  Port=2
  Fz2 : Outport  Port=3
  Fz3 : Outport  Port=4
  Fz4 : Outport  Port=5
  wires:
  In1/1 -> Kprop Constant/1
  Demux/1 -> vecZ1/1(In1)
  Demux/2 -> vecZ2/1(In1)
  Demux/3 -> vecZ3/1(In1)
  Demux/4 -> vecZ4/1(In1)
  Kprop Constant/1 -> Demux/1, Individual Fz/1
  vecZ1/1(Out1) -> Fz1/1
  vecZ2/1(Out1) -> Fz2/1
  vecZ3/1(Out1) -> Fz3/1
  vecZ4/1(Out1) -> Fz4/1

== system QuadcopterControl/Motor Conditions/Moment & Net Force/Propeller Torque  ==
  In1 : Inport
  Torque Gain (Rotor) : Gain
  vecZ : Subsystem
  zTorque : Subsystem
  Out1 : Outport
  wires:
  In1/1 -> Torque Gain (Rotor)/1
  Torque Gain (Rotor)/1 -> zTorque/1(In1)
  zTorque/1(Out1) -> vecZ/1(In1)
  vecZ/1(Out1) -> Out1/1

== system QuadcopterControl/Motor Conditions/Moment & Net Force/Propellers ==
  Rotor1 : Constant  Value=[1 -1 0.1]
  Rotor2 : Constant  Value=[1 1 0.1]
  Rotor3 : Constant  Value=[-1 1 0.1]
  Rotor4 : Constant  Value=[-1 -1 0.1]
  R1 : Outport
  R2 : Outport  Port=2
  R3 : Outport  Port=3
  R4 : Outport  Port=4
  wires:
  Rotor1/1 -> R1/1
  Rotor2/1 -> R2/1
  Rotor3/1 -> R3/1
  Rotor4/1 -> R4/1

== system QuadcopterControl/Motor Conditions/Moment & Net Force/SquareBodyRates ==
  In1 : Inport
  Abs : Abs  SaturateOnIntegerOverflow=off
  Product : Product
  Out1 : Outport
  wires:
  In1/1 -> Product/2, Abs/1
  Abs/1 -> Product/1
  Product/1 -> Out1/1

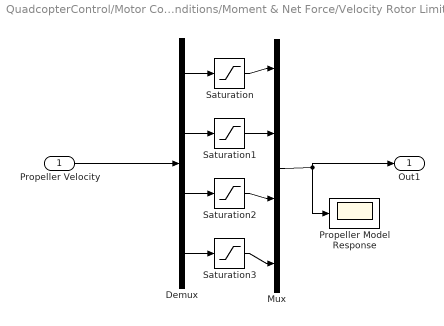
== system QuadcopterControl/Motor Conditions/Moment & Net Force/Velocity Rotor Limiter ==
  Propeller Velocity : Inport
  Demux : Demux
  Mux : Mux
  Propeller Model Response : Scope
  Saturation{,1..3} (4 alike) : Saturate  UpperLimit=0  LowerLimit=-5
  Out1 : Outport
  wires:
  Propeller Velocity/1 -> Demux/1
  Mux/1 -> Propeller Model Response/1, Out1/1
  Demux/1 -> Saturation/1
  Saturation/1 -> Mux/1
  Demux/2 -> Saturation1/1
  Saturation1/1 -> Mux/2
  Demux/3 -> Saturation2/1
  Saturation2/1 -> Mux/3
  Demux/4 -> Saturation3/1
  Saturation3/1 -> Mux/4

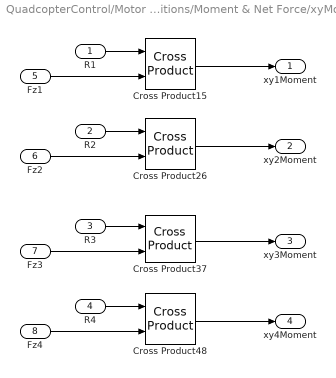
== system QuadcopterControl/Motor Conditions/Moment & Net Force/xyMoment ==
  R1 : Inport
  R2 : Inport  Port=2
  R3 : Inport  Port=3
  R4 : Inport  Port=4
  Fz1 : Inport  Port=5
  Fz2 : Inport  Port=6
  Fz3 : Inport  Port=7
  Fz4 : Inport  Port=8
  Cross Product{15,26,37,48} (4 alike) : matrix_library/Cross Product
  xy1Moment : Outport
  xy2Moment : Outport  Port=2
  xy3Moment : Outport  Port=3
  xy4Moment : Outport  Port=4
  wires:
  R4/1 -> Cross Product48/1
  Fz4/1 -> Cross Product48/2
  Fz3/1 -> Cross Product37/2
  R3/1 -> Cross Product37/1
  R2/1 -> Cross Product26/1
  Fz2/1 -> Cross Product26/2
  Fz1/1 -> Cross Product15/2
  R1/1 -> Cross Product15/1
  Cross Product15/1 -> xy1Moment/1
  Cross Product26/1 -> xy2Moment/1
  Cross Product37/1 -> xy3Moment/1
  Cross Product48/1 -> xy4Moment/1

== system QuadcopterControl/Motor Conditions/Rotor Correction/Rotor Allocation ==
  Magnitude : Gain  Gain=-1
  Mass : Gain
  Rotor Coefficient : Gain  Gain=9.81/4
  RotorArray : Constant  Value=[1;1;1;1]
  Out1 : Outport
  wires:
  RotorArray/1 -> Mass/1
  Mass/1 -> Magnitude/1
  Magnitude/1 -> Rotor Coefficient/1
  Rotor Coefficient/1 -> Out1/1

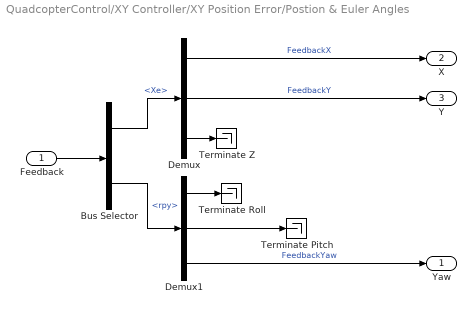
== system QuadcopterControl/XY Controller/XY Position Error/Postion & Euler Angles  ==
  Feedback : Inport
  Bus Selector : BusSelector  OutputSignals=Xe,rpy
  Demux : Demux  Outputs=3
  Demux1 : Demux  Outputs=3
  Terminate Pitch : Terminator
  Terminate Roll : Terminator
  Terminate Z : Terminator
  Yaw : Outport
  X : Outport  Port=2
  Y : Outport  Port=3
  wires:
  Feedback/1 -> Bus Selector/1
  Bus Selector/1 -> Demux/1  "<Xe>"
  Demux/1 -> X/1  "FeedbackX"
  Demux/2 -> Y/1  "FeedbackY"
  Demux/3 -> Terminate Z/1
  Bus Selector/2 -> Demux1/1  "<rpy>"
  Demux1/1 -> Terminate Roll/1
  Demux1/2 -> Terminate Pitch/1
  Demux1/3 -> Yaw/1  "FeedbackYaw"

== system QuadcopterControl/Motor Conditions/Moment & Net Force/F_BodyZ/vecZ ==
  InputFz : Inport
  ArrayZ : Constant  Value=[0; 0; 1]
  Product : Product
  OutputFz : Outport
  wires:
  Product/1 -> OutputFz/1
  InputFz/1 -> Product/2
  ArrayZ/1 -> Product/1

== system QuadcopterControl/Motor Conditions/Moment & Net Force/Propeller Forces/vecZ1 ==
  In1 : Inport
  ArrayZ : Constant  Value=[0;0;1]
  Product : Product
  Out1 : Outport
  wires:
  ArrayZ/1 -> Product/1
  Product/1 -> Out1/1
  In1/1 -> Product/2

== system QuadcopterControl/Motor Conditions/Moment & Net Force/Propeller Forces/vecZ2 ==
  In1 : Inport
  ArrayZ : Constant  Value=[0; 0; 1]
  Product : Product
  Out1 : Outport
  wires:
  ArrayZ/1 -> Product/1
  In1/1 -> Product/2
  Product/1 -> Out1/1

== system QuadcopterControl/Motor Conditions/Moment & Net Force/Propeller Forces/vecZ3 ==
  In1 : Inport
  ArrayZ : Constant  Value=[0; 0; 1]
  Product : Product
  Out1 : Outport
  wires:
  In1/1 -> Product/2
  Product/1 -> Out1/1
  ArrayZ/1 -> Product/1

== system QuadcopterControl/Motor Conditions/Moment & Net Force/Propeller Forces/vecZ4 ==
  In1 : Inport
  ArrayZ : Constant  Value=[0; 0; 1]
  Product : Product
  Out1 : Outport
  wires:
  In1/1 -> Product/2
  Product/1 -> Out1/1
  ArrayZ/1 -> Product/1

== system QuadcopterControl/Motor Conditions/Moment & Net Force/Propeller Torque /vecZ ==
  In1 : Inport
  ArrayZ : Constant  Value=[0;0;1]
  Product : Product
  Out1 : Outport
  wires:
  Product/1 -> Out1/1
  In1/1 -> Product/2
  ArrayZ/1 -> Product/1

== system QuadcopterControl/Motor Conditions/Moment & Net Force/Propeller Torque /zTorque ==
  In1 : Inport
  Constant : Constant  Value=[-1; 1; -1; 1]
  Product : Product
  Sum of Elements : Sum  Inputs=+
  Out1 : Outport
  wires:
  Constant/1 -> Product/1
  In1/1 -> Product/2
  Product/1 -> Sum of Elements/1
  Sum of Elements/1 -> Out1/1
